simulink model "CLIKsecordine"  (R2024a)
settings: Solver=VariableStepAuto  StartTime=0.0  StopTime=100  RelTol=1e-3
values from neighbouring files (symbols this model uses):
  Kd = diag([108 68 58 200])    [TRAIETTORIA.m]    (also in traiettoriafperfettadefinitiva1.m)
  Kp = diag([13 13 11 1000])    [TRAIETTORIA.m]    (also in traiettoriafperfettadefinitiva1.m)
undefined symbols (not defined in the file or in its folder): DiscIntNeverNeededParam
settings Model: Creator=ThinkPad  LastModifiedBy=UTENTE
settings ModelReferenceCC: EnableRefExpFcnMdlSchedulingChecks=on
settings RTWCC: GPUComputeCapability=3.5

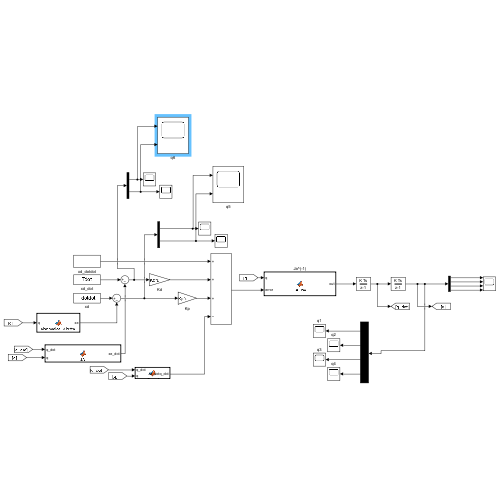
[thumbnail: Simulink's stored preview of the top-level diagram]
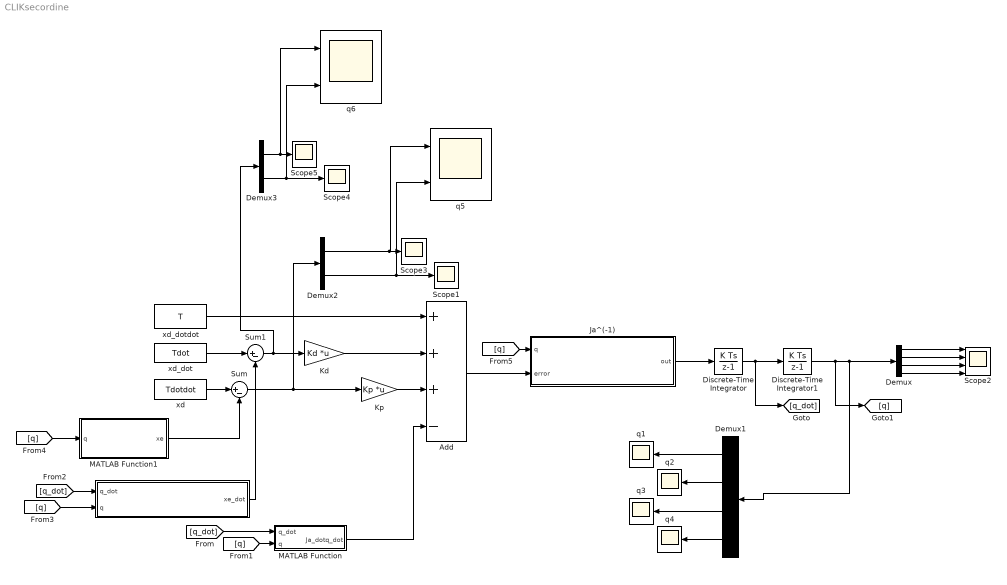
== system CLIKsecordine ==
  "  " : MATLAB Function  TreatAsAtomicUnit=on
  Add : Sum  Inputs=+++-
  Demux : Demux
  Demux1 : Demux
  Demux2 : Demux  Outputs=[3 1]
  Demux3 : Demux  Outputs=[3 1]
  Discrete-Time Integrator : DiscreteIntegrator  InitialCondition=[0 0 0 0]'  SampleTime=0.001  ICPrevOutput=DiscIntNeverNeededParam  ICPrevScaledInput=DiscIntNeverNeededParam
  Discrete-Time Integrator1 : DiscreteIntegrator  InitialCondition=[pi/4,pi/6,pi/5,0.5]'  SampleTime=0.001  ICPrevOutput=DiscIntNeverNeededParam  ICPrevScaledInput=DiscIntNeverNeededParam
  Ja^(-1) : MATLAB Function  TreatAsAtomicUnit=on
  Kd : Gain  Gain=Kd  Multiplication=Matrix(K*u)
  Kp : Gain  Gain=Kp  Multiplication=Matrix(K*u)
  MATLAB Function : MATLAB Function  TreatAsAtomicUnit=on
  MATLAB Function1 : MATLAB Function  TreatAsAtomicUnit=on
  Scope{1,3..5} (4 alike) : Scope
  Scope2 : Scope  NumInputPorts=4
  Sum : Sum  Inputs=|+-
  Sum1 : Sum  Inputs=|+-
  q{1..4} (4 alike) : Scope
  q5 : Scope  NumInputPorts=2
  q6 : Scope  NumInputPorts=2
  xd : FromWorkspace  VariableName=Tdotdot
  xd_dot : FromWorkspace  VariableName=Tdot
  xd_dotdot : FromWorkspace  VariableName=T
  wires:
  Demux1/2 -> q2/1
  xd_dot/1 -> Sum1/1
  Demux/4 -> Scope2/4
  Kd/1 -> Add/2
  Demux1/3 -> q3/1
  MATLAB Function1/1(xe) -> Sum/2
  Demux1/1 -> q1/1
  Discrete-Time Integrator/1 -> [q_dot], Discrete-Time Integrator1/1
  MATLAB Function/1(Ja_dotq_dot) -> Add/4
  Sum/1 -> Kp/1, Demux2/1
  xd/1 -> Sum/1
  Kp/1 -> Add/3
  Ja^(-1)/1(out) -> Discrete-Time Integrator/1
  Demux/3 -> Scope2/3
  Add/1 -> Ja^(-1)/2(error)
  Demux/1 -> Scope2/1
  xd_dotdot/1 -> Add/1
  "  "/1(xe_dot) -> Sum1/2
  Demux1/4 -> q4/1
  Demux/2 -> Scope2/2
  Discrete-Time Integrator1/1 -> [q], Demux/1, Demux1/1
  [q_dot] -> MATLAB Function/1(q_dot)
  [q] -> MATLAB Function/2(q)
  [q] -> "  "/2(q)
  [q_dot] -> "  "/1(q_dot)
  [q] -> MATLAB Function1/1(q)
  [q] -> Ja^(-1)/1(q)
  Demux2/2 -> Scope1/1, q5/2
  Demux2/1 -> q5/1, Scope3/1
  Demux3/2 -> Scope4/1, q6/2
  Demux3/1 -> q6/1, Scope5/1
  Sum1/1 -> Demux3/1, Kd/1

== matlab function CLIKsecordine/Ja^(-1) ==
  data: q input; out output; error input
function out= JA_inv(q,error)

J=[-0.5*sin(q(1))-0.5*sin(q(1)+q(2)) -0.5*sin(q(1)+q(2)) 0 0;
    0.5*cos(q(1))+0.5*cos(q(1)+q(2)) 0.5*cos(q(1)+q(2)) 0 0;
    0 0 -1 0;
    1 1 0 -1];

J_inv=inv(J);

 inverse_Jacobian=J_inv;
 out = inverse_Jacobian*error;
end

== matlab function CLIKsecordine/   ==
  data: q_dot input; q input; xe_dot output
function xe_dot = JA(q_dot, q)

J=[-0.5*sin(q(1))-0.5*sin(q(1)+q(2)) -0.5*sin(q(1)+q(2)) 0 0;
    0.5*cos(q(1))+0.5*cos(q(1)+q(2)) 0.5*cos(q(1)+q(2)) 0 0;
    0 0 -1 0;
    1 1 0 -1];
xe_dot=J*q_dot;
end

== matlab function CLIKsecordine/MATLAB Function ==
  data: q_dot input; q input; Ja_dotq_dot output
function Ja_dotq_dot = JA_dot(q_dot, q)
J_dot=[-0.5*cos(q(1))*q_dot(1)-0.5*cos(q(1)+q(2))*(q_dot(1)+q_dot(2)) -0.5*cos(q(1)+q(2))*(q_dot(1)+q_dot(2)) 0 0;
    -0.5*sin(q(1))*q_dot(1)-0.5*sin(q(1)+q(2))*(q_dot(1)+q_dot(2)) -0.5*sin(q(1)+q(2))*(q_dot(1)+q_dot(2)) 0 0;
    0 0 0 0;
    0 0 0 0];
Ja_dotq_dot=J_dot*q_dot;
end

== matlab function CLIKsecordine/MATLAB Function1 ==
  data: q input; xe output
function xe = cinematica_diretta(q)
% T_4_0=[cos(q(4))*(cos(q(1))*cos(q(2))-sin(q1)*sin(q2))+sin(q(4))*(cos(q1)*sin(q(2))+cos(q(2))*sin(q(1)))   cos(q(4))*(cos(q(1))*sin(q(2))+cos(q(2))*sin(q(1)))-sin(q(4))*(cos(q(1))*cos(q(2))-sin(q(1))*sin(q(2)))  0 cos(q(1))/2+(cos(q(1))*cos(q(2)))/2-(sin(q(1))*sin(q(2)))/2;
%         cos(q(4))*(cos(q(1))*sin(q(2))+cos(q(2))*sin(q(1)))-sin(q(4))*(cos(q(1))*cos(q(2))-sin(q(1))*sin(q(2))) -cos(q(4))*(cos(q(1))*cos(q(2))-sin(q(1))*sin(q(2)))-sin(q(4))*(cos(q(1))*sin(q(2))+cos(q(2))*sin(q(1)))  0 sin(q(1))/2+(cos(q(1))*sin(q(2)))/2+(cos(q(2))*sin(q(2)))/2;
%                       0                                                      0                    -1                                                1-q(3);
%         0                                       0                                         0                                                                                                                                      1];

x_e=[0.5*cos(q(1))+0.5*cos(q(1)+q(2));
    0.5*sin(q(1))+0.5*sin(q(1)+q(2));
        1-q(3);
        q(1)+q(2)-q(4)];
xe=x_e;
end
